simulink model "Houghline_LIB"  (R2016a)
settings: Solver=VariableStepAuto  StartTime=0.0  StopTime=1  RelTol=1e-3
undefined symbols (not defined in the file): gray, Rec, SDTV, strel
libraries: visiontransforms x3, visionmorphops x2, visiontextngfix x2, visionanalysis x2, visionconversions x1, visionstatistics x1, visionsources x1
settings Model: Creator=Yewly  LastModifiedBy=Yewly
settings GRTTargetCC: GeneratePreprocessorConditionals=Use local settings

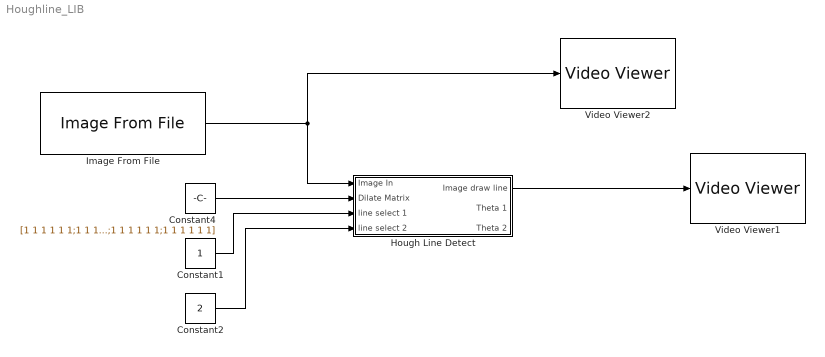
== system Houghline_LIB ==
  Constant1 : Constant  OutDataTypeStr=double
  Constant2 : Constant  Value=2  OutDataTypeStr=double
  Constant4 : Constant  Value=[1 1 1 1 1 1;1 1 1 1 1 1;1 1 1 1 1 1;1 1 1 1 1 1;1 1 1 1 1 1;1 1 1 1 1 1]  OutDataTypeStr=boolean
  "Hough Line Detect " : Subsystem
  Image From File : visionsources/Image From File  Tag=vipblks_nd  FileName=road.jpg  imagePorts=One multidimensional signal  Ts=1  ImageDataType=Inherit from input image  Signed=on  WordLength=16  sdImageDataType=uint(8)  FractionLengthMode=User-defined  FractionLength=15  OutPortLabels=R|G|B
  Video Viewer1 : VideoViewer  colormapValue=gray(256)  FigPos=[366.6 729.2 714.4 445.6]
  Video Viewer2 : VideoViewer  colormapValue=gray(256)  FigPos=[25.8 770.8 714.4 445.6]
  wires:
  Constant4/1 -> "Hough Line Detect "/2("Dilate Matrix ")
  "Hough Line Detect "/1("Image draw line ") -> Video Viewer1/1
  Constant1/1 -> "Hough Line Detect "/3(line select 1)
  Constant2/1 -> "Hough Line Detect "/4(line select 2)
  Image From File/1 -> "Hough Line Detect "/1(Image In), Video Viewer2/1

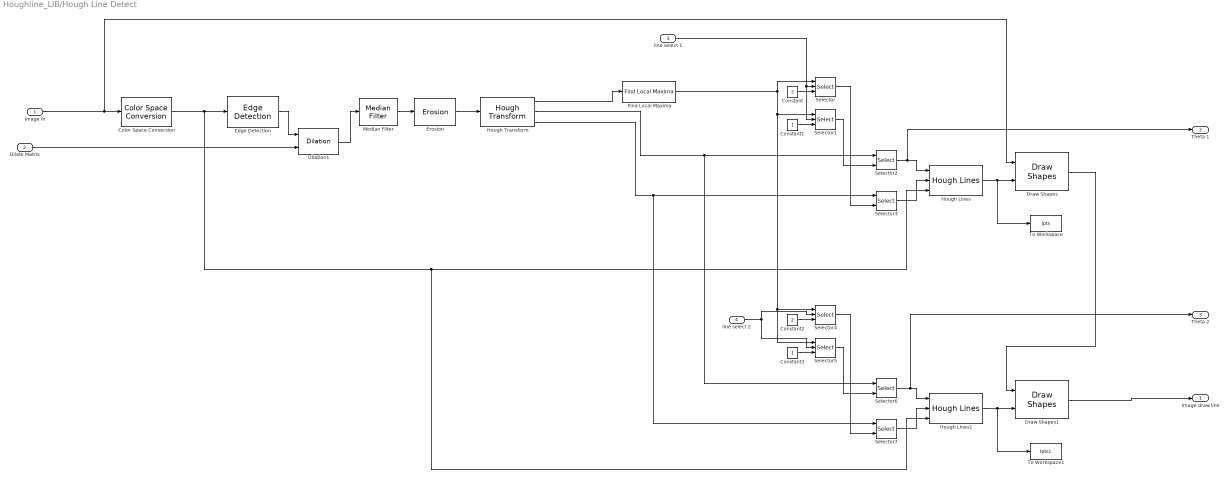
== system Houghline_LIB/Hough Line Detect  ==
  Image In : Inport
  "Dilate Matrix " : Inport  Port=2
  line select 1 : Inport  Port=3
  line select 2 : Inport  Port=4
  Color Space Conversion : visionconversions/Color Space  Conversion  conversion=Obsolete  conversionActive=R'G'B' to intensity  wp_str=D65  rec=Rec. 601 (SDTV)  sys=1125/60/2:1  imagePorts=One multidimensional signal
  Constant : Constant  Value=2
  Constant1 : Constant
  Constant2 : Constant  Value=2
  Constant3 : Constant
  Dilation1 : visionmorphops/Dilation  nhoodsrc=Input port  strel=[1 1 1 1 1 1;1 1 1 1 1 1;1 1 1 1 1 1;1 1 1 1 1 1;1 1 1 1 1 1;1 1 1 1 1 1]
  Draw Shapes : visiontextngfix/Draw Shapes  shape=Lines  fill=off  lineWidth=10  fillClrSource=Specify via dialog  display=User-specified value  intensity=200  color=[200 255 50]  opacity=0.6  viewport=Entire image  antialiasing=off  inType=Obsolete  imagePorts=One multidimensional signal  prodOutputMode=Binary point scaling  prodOutputWordLength=32  prodOutputFracLength=14  memoryMode=Specify word length  memoryWordLength=16  memoryFracLength=14  roundingMode=Floor  overflowMode=off
  Draw Shapes1 : visiontextngfix/Draw Shapes  shape=Lines  fill=off  lineWidth=10  fillClrSource=Specify via dialog  display=User-specified value  intensity=200  color=[200 255 50]  opacity=0.6  viewport=Entire image  antialiasing=off  inType=Obsolete  imagePorts=One multidimensional signal  prodOutputMode=Binary point scaling  prodOutputWordLength=32  prodOutputFracLength=14  memoryMode=Specify word length  memoryWordLength=16  memoryFracLength=14  roundingMode=Floor  overflowMode=off
  Edge Detection : visionanalysis/Edge Detection  method=Sobel  outputType=Binary image  userDefinedThreshold=off  thresholdSource=Input port  threshold=20  thresholdTuning=4  edgeThinning=on  threshold_canny=[0.25 0.60]  autoPercent=70  sigma=1  prodOutputMode=Binary point scaling  prodOutputWordLength=32  prodOutputFracLength=8  roundingMode=Floor  overflowMode=off
  Erosion : visionmorphops/Erosion  nhoodsrc=Specify via dialog  strel=strel('square',12)
  Find Local Maxima : visionstatistics/Find Local Maxima  num_peaks=5  nhood_size=[5 7]  src_thresh=Obsolete9b  src_thresh_inuse=Specify via dialog  threshold=10  inputIsHough=on  dt_peak=uint32  isOutVarDim=on  dt_count=uint32
  Hough Lines : visiontransforms/Hough Lines  sineCompMethod=Trigonometric function  thetaRes=pi/180  firstCoeffMode=Specify word length  firstCoeffWordLength=16  firstCoeffFracLength=15  prodOutputMode=Binary point scaling  prodOutputWordLength=32  prodOutputFracLength=16  roundingMode=Nearest  overflowMode=on
  Hough Lines1 : visiontransforms/Hough Lines  sineCompMethod=Trigonometric function  thetaRes=pi/180  firstCoeffMode=Specify word length  firstCoeffWordLength=16  firstCoeffFracLength=15  prodOutputMode=Binary point scaling  prodOutputWordLength=32  prodOutputFracLength=16  roundingMode=Nearest  overflowMode=on
  Hough Transform : visiontransforms/Hough Transform  theta_res=pi/360  rho_res=1  out_theta_rho=on  outdtmode=double  firstCoeffMode=Binary point scaling  firstCoeffWordLength=16  firstCoeffFracLength=14  secondCoeffMode=Binary point scaling  secondCoeffWordLength=32  secondCoeffFracLength=16  outputMode=Binary point scaling  outputWordLength=16  outputFracLength=0  accumMode=Binary point scaling  accumWordLength=32  accumFracLength=20  prodOutputMode=Binary point scaling  prodOutputWordLength=32  prodOutputFracLength=20  memoryMode=Binary point scaling  memoryWordLength=32  memoryFracLength=16  roundingMode=Nearest  overflowMode=on
  Median Filter : visionanalysis/Median Filter  nghbood=[3 3]  outSize=Same as input port I  padType=Symmetric  padSrc=Specify via dialog  padVal=0  roundingMode=Floor  overflowMode=off
  Selector : Selector  NumberOfDimensions=2  InputPortWidth=2  IndexOptions=Index vector (port),Index vector (port)  Indices=1,1  OutputSizes=1,1
  Selector1 : Selector  NumberOfDimensions=2  InputPortWidth=2  IndexOptions=Starting index (port),Index vector (port)  Indices=1,1  OutputSizes=1,1
  Selector{2..3,6..7} (4 alike) : Selector  NumberOfDimensions=2  InputPortWidth=3  IndexOptions=Select all,Index vector (port)  Indices=[1 3],1  OutputSizes=1,1
  Selector4 : Selector  NumberOfDimensions=2  InputPortWidth=2  IndexOptions=Index vector (port),Index vector (port)  Indices=2,1  OutputSizes=1,1
  Selector5 : Selector  NumberOfDimensions=2  InputPortWidth=2  IndexOptions=Index vector (port),Index vector (port)  Indices=2,1  OutputSizes=1,1
  To Workspace : ToWorkspace  VariableName=lpts  SampleTime=-1
  To Workspace1 : ToWorkspace  VariableName=lpts1  SampleTime=-1
  "Image draw line " : Outport
  Theta 1 : Outport  Port=2
  Theta 2 : Outport  Port=3
  wires:
  Image In/1 -> Draw Shapes/1, Color Space Conversion/1
  Selector5/1 -> Selector6/2
  Draw Shapes1/1 -> "Image draw line "/1
  Constant1/1 -> Selector1/3
  Constant3/1 -> Selector5/3
  Selector3/1 -> Hough Lines/2
  Hough Transform/3 -> Selector7/1, Selector3/1
  Selector4/1 -> Selector7/2
  Find Local Maxima/1 -> Selector5/1, Selector4/1, Selector1/1, Selector/1
  Hough Lines/1 -> To Workspace/1, Draw Shapes/2
  Hough Transform/1 -> Find Local Maxima/1
  Edge Detection/1 -> Dilation1/1
  Selector7/1 -> Hough Lines1/2
  Hough Lines1/1 -> To Workspace1/1, Draw Shapes1/2
  Selector1/1 -> Selector2/2
  Constant2/1 -> Selector4/3
  Color Space Conversion/1 -> Hough Lines1/3, Hough Lines/3, Edge Detection/1
  Hough Transform/2 -> Selector6/1, Selector2/1
  Dilation1/1 -> Median Filter/1
  Selector/1 -> Selector3/2
  Erosion/1 -> Hough Transform/1
  Draw Shapes/1 -> Draw Shapes1/1
  Median Filter/1 -> Erosion/1
  "Dilate Matrix "/1 -> Dilation1/2
  Selector2/1 -> Theta 1/1, Hough Lines/1
  Selector6/1 -> Theta 2/1, Hough Lines1/1
  line select 1/1 -> Selector1/2, Selector/2
  Constant/1 -> Selector/3
  line select 2/1 -> Selector5/2, Selector4/2
